simulink model "NetworkModelIntermediateIntersectionCRCA"  (R2018b)
settings: Solver=VariableStepAuto  StartTime=0.0  StopTime=10.0  RelTol=1e-3
values from neighbouring files (symbols this model uses):
  Ax = [0 1  0   0 ... (first row only)    [DroneSubsystemModelling.m]
  Ay = [0 1  0   0 ... (first row only)    [DroneSubsystemModelling.m]
  Bx = [0;0;0;b1]    [DroneSubsystemModelling.m]
  By = [0;0;0;b2]    [DroneSubsystemModelling.m]
  ConflictDrone1andDrone2 = ControlDetectionFunction(tout,PositionXDrone1TEST, PositionYDrone1TEST, PositionXDrone2TEST, PositionYDrone2TEST, ConflictDrone1andDrone2)    [ConflictDetectionTEST.m]
  ConflictDrone1andDrone3 = ControlDetectionFunction(tout,PositionXDrone1TEST, PositionYDrone1TEST, PositionXDrone3TEST, PositionYDrone3TEST, ConflictDrone1andDrone3)    [ConflictDetectionTEST.m]
  ConflictDrone1andDrone4 = ControlDetectionFunction(tout,PositionXDrone1TEST, PositionYDrone1TEST, PositionXDrone4TEST, PositionYDrone4TEST, ConflictDrone1andDrone4)    [ConflictDetectionTEST.m]
  ConflictDrone2andDrone3 = ControlDetectionFunction(tout,PositionXDrone2TEST, PositionYDrone2TEST, PositionXDrone3TEST, PositionYDrone3TEST, ConflictDrone2andDrone3)    [ConflictDetectionTEST.m]
  ConflictDrone2andDrone4 = ControlDetectionFunction(tout,PositionXDrone2, PositionYDrone2, PositionXDrone4, PositionYDrone4, ConflictDrone2andDrone4)    [ConflictDetection.m]    (also in ConflictDetectionTEST.m = ControlDetectionFunction(tout,PositionXDrone2TEST, PositionY)
  ConflictDrone3andDrone4 = ControlDetectionFunction(tout,PositionXDrone3TEST, PositionYDrone3TEST, PositionXDrone4TEST, PositionYDrone4TEST, ConflictDrone3andDrone4)    [ConflictDetectionTEST.m]
  ConflictDrone7andDrone8 = ControlDetectionFunction(tout,PositionXDrone7TEST, PositionYDrone7TEST, PositionXDrone8TEST, PositionYDrone8TEST, ConflictDrone7andDrone8)    [ConflictDetectionTEST.m]
  Cpx = [1 0 0 0]    [DroneSubsystemModelling.m]
  Cpy = [1 0 0 0]    [DroneSubsystemModelling.m]
  Cvx = [0 1 0 0]    [DroneSubsystemModelling.m]
  Cvy = [0 1 0 0]    [DroneSubsystemModelling.m]
  theta1 = -180    [MotionModelling.m]
  theta2 = -3*180/4    (= -135)    [MotionModelling.m]
  theta3 = -2*180/4    (= -90)    [MotionModelling.m]
  theta4 = -180/4    (= -45)    [MotionModelling.m]
  theta5 = 2*180    (= 360)    [MotionModelling.m]
  theta6 = 180/4    (= 45)    [MotionModelling.m]
  theta7 = 2*180/4    (= 90)    [MotionModelling.m]
  theta8 = 3*180/4    (= 135)    [MotionModelling.m]
  VelocityStarX1 = vx10    [MotionModelling.m]
  VelocityStarX2 = vx20    [MotionModelling.m]
  VelocityStarX3 = vx30    [MotionModelling.m]
  VelocityStarX4 = vx40    [MotionModelling.m]
  VelocityStarX5 = vx50    [MotionModelling.m]
  VelocityStarX6 = vx60    [MotionModelling.m]
  VelocityStarX7 = vx70    [MotionModelling.m]
  VelocityStarX8 = vx80    [MotionModelling.m]
  VelocityStarY1 = vy10    [MotionModelling.m]
  VelocityStarY2 = vy20    [MotionModelling.m]
  VelocityStarY3 = vy30    [MotionModelling.m]
  VelocityStarY4 = vy40    [MotionModelling.m]
  VelocityStarY5 = vy50    [MotionModelling.m]
  VelocityStarY6 = vy60    [MotionModelling.m]
  VelocityStarY7 = vy70    [MotionModelling.m]
  VelocityStarY8 = vy80    [MotionModelling.m]
  X10 = [x10 vx10 0 0]'    [MotionModelling.m]
  X20 = [x20 vx20 0 0]'    [MotionModelling.m]
  X30 = [x30 vx30 0 0]'    [MotionModelling.m]
  X40 = [x40 vx40 0 0]'    [MotionModelling.m]
  X50 = [x50 vx50 0 0]'    [MotionModelling.m]
  X60 = [x60 vx60 0 0]'    [MotionModelling.m]
  X70 = [x70 vx70 0 0]'    [MotionModelling.m]
  X80 = [x80 vx80 0 0]'    [MotionModelling.m]
  Y10 = [y10 vy10 0 0]'    [MotionModelling.m]
  Y20 = [y20 vy20 0 0]'    [MotionModelling.m]
  Y30 = [y30 vy30 0 0]'    [MotionModelling.m]
  Y40 = [y40 vy40 0 0]'    [MotionModelling.m]
  Y50 = [y50 vy50 0 0]'    [MotionModelling.m]
  Y60 = [y60 vy60 0 0]'    [MotionModelling.m]
  Y70 = [y70 vy70 0 0]'    [MotionModelling.m]
  Y80 = [y80 vy80 0 0]'    [MotionModelling.m]
undefined symbols (not defined in the file or in its folder): ConflictDrone5andDrone6, K
libraries: simulink x16
(part 1 of 2)
settings Model: Creator=CowUser  LastModifiedBy=CowUser
settings ConfigComp: DVTestSuiteOptimization=CombinedObjectives (Nonlinear Extended)  DVDetectOutOfBounds=on

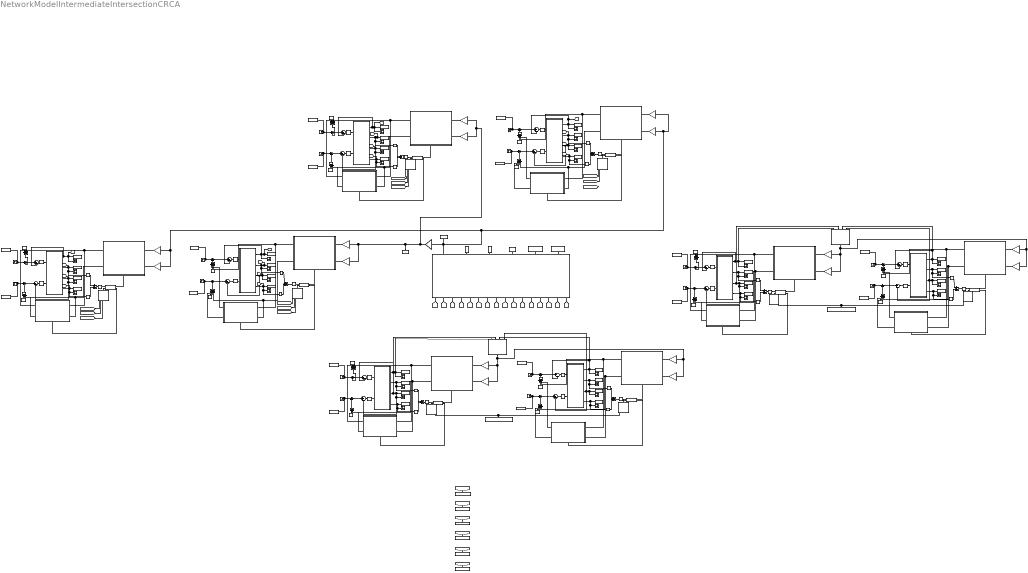
== system NetworkModelIntermediateIntersectionCRCA ==
  note: Drone 4
  note: Intermediate Intersection
      | (based on closure rate and closure angle)
      |
      | Right Hand Rule
  note: Drone 2
  note: Drone 5
  note: Drone 6
  note: Sample
  note: Drone 1
  note: Drone 3
  note: Drone 7
  note: Sample
  note: Drone 8
  note: Sample 4
  note: Sample 2
  note: Sample 6
  note: Sample 3
  note: Sample 5
  note: Sample 1
  Add{1..4,7,10..16,19..22} (16 alike) : Sum  Inputs=+++
  Add{5..6,8..9,17..18,23..24} (8 alike) : Sum
  Constant{1..4,6..8,10..14,16..19} (16 alike) : Constant  Value=0
  Constant20 : Constant  Value=ConflictDrone7andDrone8
  Constant25 : Constant  Value=ConflictDrone1andDrone3
  Constant26 : Constant  Value=ConflictDrone1andDrone2
  Constant27 : Constant  Value=ConflictDrone1andDrone4
  Constant28 : Constant  Value=ConflictDrone2andDrone4
  Constant29 : Constant  Value=ConflictDrone3andDrone4
  Constant30 : Constant  Value=ConflictDrone2andDrone3  VectorParams1D=off
  Constant5 : Constant  Value=ConflictDrone5andDrone6
  Drone1 Subsystem : Subsystem
  Drone2 Subsystem : Subsystem
  Drone2 Subsystem3 : Subsystem
  Drone3 Subsystem : Subsystem
  Drone4 Subsystem : Subsystem
  Drone4 Subsystem3 : Subsystem
  Drone5 Subsystem : Subsystem
  Drone6 Subsystem : Subsystem
  Gain : Gain  Gain=K
  Gain1 : Gain  Gain=-sind (theta4)
  Gain10 : Gain  Gain=cosd (theta1)
  Gain11 : Gain  Gain=-cosd (theta3)
  Gain12 : Gain  Gain=sind (theta1)
  Gain13 : Gain  Gain=-sind (theta8)
  Gain14 : Gain  Gain=cosd (theta7)
  Gain15 : Gain  Gain=-cosd (theta8)
  Gain16 : Gain  Gain=sind (theta7)
  Gain2 : Gain  Gain=cosd (theta2)
  Gain3 : Gain  Gain=-cosd (theta4)
  Gain4 : Gain  Gain=sind (theta2)
  Gain5 : Gain  Gain=-sind (theta6)
  Gain6 : Gain  Gain=cosd (theta5)
  Gain7 : Gain  Gain=-cosd (theta6)
  Gain8 : Gain  Gain=sind (theta5)
  Gain9 : Gain  Gain=-sind (theta3)
  If Action Subsystem1 : Subsystem  TreatAsAtomicUnit=on
  If Action Subsystem2 : Subsystem  TreatAsAtomicUnit=on
  If Action Subsystem3 : Subsystem  TreatAsAtomicUnit=on
  If Action Subsystem4 : Subsystem  TreatAsAtomicUnit=on
  If Action Subsystem5 : Subsystem  TreatAsAtomicUnit=on
  If Action Subsystem6 : Subsystem  TreatAsAtomicUnit=on
  If Action Subsystem7 : Subsystem  TreatAsAtomicUnit=on
  If Action Subsystem8 : Subsystem  TreatAsAtomicUnit=on
  If{1..8} (8 alike) : If  NumInputs=2  IfExpression=(u1 <= R)&(u2 == 1)  ElseIfExpressions=(u1 > R)&(u2 == 1)  ShowElse=off
  MATLAB Function1 : MATLAB Function  TreatAsAtomicUnit=on
  MATLAB Function2 : MATLAB Function  TreatAsAtomicUnit=on
  MATLAB Function3 : MATLAB Function  TreatAsAtomicUnit=on
  OR{1..8} (8 alike) : Logic  Operator=OR  Inputs=7  IconShape=distinctive  AllPortsSameDT=off  OutDataTypeStr='double'
  PID Controller{1..16} (16 alike) : simulink/Continuous/PID Controller  Controller=PID  Form=Parallel  TimeDomain=Continuous-time  SampleTime=-1  IntegratorMethod=Forward Euler  FilterMethod=Forward Euler  ControllerParametersSource=internal  P=1.97139727738968e-05  I=1.5233344900537e-08  D=0.00566857635684116  UseFilter=on  N=15.1370363747334  TunerSelectOption=Transfer Function Based (PID Tuner App)  InitialConditionSource=internal  InitialConditionForIntegrator=0  InitialConditionForFilter=0  DifferentiatorICPrevScaledInput=0  ExternalReset=none  TrackingMode=off  Kt=1  LimitOutput=off  UpperSaturationLimit=inf  LowerSaturationLimit=-inf  LinearizeAsGain=on  AntiWindupMode=none  Kb=1  POutMin=[]  POutMax=[]  IOutMin=[]  IOutMax=[]  DOutMin=[]  DOutMax=[]  NOutMin=[]  NOutMax=[]  SumOutMin=[]  SumOutMax=[]  SaturationOutMin=[]  SaturationOutMax=[]  PParamMin=[]  PParamMax=[]  IParamMin=[]  IParamMax=[]  DParamMin=[]  DParamMax=[]  NParamMin=[]  NParamMax=[]  KbParamMin=[]  KbParamMax=[]  KtParamMin=[]  KtParamMax=[]  KbOutMin=[]  KbOutMax=[]  KtOutMin=[]  KtOutMax=[]  IntegratorOutMin=[]  IntegratorOutMax=[]  FilterOutMin=[]  FilterOutMax=[]  SumI1OutMin=[]  SumI1OutMax=[]  SumI2OutMin=[]  SumI2OutMax=[]  SumI3OutMin=[]  SumI3OutMax=[]  SumI4OutMin=[]  SumI4OutMax=[]  SumDOutMin=[]  SumDOutMax=[]  DifferentiatorOutMin=[]  DifferentiatorOutMax=[]  FilterDiffOutCoefMin=[]  FilterDiffOutCoefMax=[]  ReciprocalOutMin=[]  ReciprocalOutMax=[]  SumDenOutMin=[]  SumDenOutMax=[]  SumNumOutMin=[]  SumNumOutMax=[]  DivideOutMin=[]  DivideOutMax=[]  IntegratorContinuousStateAttributes=''  IntegratorStateMustResolveToSignalObject=off  IntegratorRTWStateStorageClass=Auto  FilterContinuousStateAttributes=''  FilterStateMustResolveToSignalObject=off  FilterRTWStateStorageClass=Auto  ParallelPVariant=InternalParameters  IdealPVariant=Disabled  IVariant=InternalParameters  DVariant=InternalParameters  IntegratorVariant=Continuous  SatVariant=Disabled  AWVariant=Passthrough  PCopyVariant=Disabled  TRVariant=Disabled  FdbkBlocksVariant=Forward  IdealPFdbkVariant=Disabled  SatFdbkVariant=Disabled  DerivativeFilterVariant=ContFilter  NVariant=InternalParameters  NCopyVariant=Disabled  FilterICVariant=InternalICsFilter  IntegratorICVariant=InternalICs  ExternalResetVariant=Disabled  TRSumVariant=Passthrough  SumFdbkVariant=Disabled  SumVariant=Sum_PID
  PositionXDrone{1,3,5..8,11,44} (8 alike) : Scope
  PositionYDrone{1,3,5..8,11,44} (8 alike) : Scope
  Sqrt{1..8} (8 alike) : Sqrt  SaturateOnIntegerOverflow=on
  Square{1..16} (16 alike) : Math  Operator=square  SaturateOnIntegerOverflow=on
  Step 1 : Step  Time=0  After=VelocityStarX5  SampleTime=0
  Step 10 : Step  Time=0  After=VelocityStarY1  SampleTime=0
  Step 11 : Step  Time=0  After=VelocityStarX3  SampleTime=0
  Step 12 : Step  Time=0  After=VelocityStarY3  SampleTime=0
  Step 13 : Step  Time=0  After=VelocityStarX7  SampleTime=0
  Step 14 : Step  Time=0  After=VelocityStarY7  SampleTime=0
  Step 15 : Step  Time=0  After=VelocityStarX8  SampleTime=0
  Step 16 : Step  Time=0  After=VelocityStarY8  SampleTime=0
  Step 2 : Step  Time=0  After=VelocityStarY5  SampleTime=0
  Step 3 : Step  Time=0  After=VelocityStarX2  SampleTime=0
  Step 4 : Step  Time=0  After=VelocityStarY2  SampleTime=0
  Step 5 : Step  Time=0  After=VelocityStarX4  SampleTime=0
  Step 6 : Step  Time=0  After=VelocityStarY4  SampleTime=0
  Step 7 : Step  Time=0  After=VelocityStarX6  SampleTime=0
  Step 8 : Step  Time=0  After=VelocityStarY6  SampleTime=0
  Step 9 : Step  Time=0  After=VelocityStarX1  SampleTime=0
  Sum{1..32} (32 alike) : Sum  Inputs=|+-
  Switch Case Action Subsystem : Subsystem  TreatAsAtomicUnit=on
  Switch Case Action Subsystem1 : Subsystem  TreatAsAtomicUnit=on
  Switch Case Action Subsystem2 : Subsystem  TreatAsAtomicUnit=on
  Switch Case Action Subsystem3 : Subsystem  TreatAsAtomicUnit=on
  Switch Case Action Subsystem4 : Subsystem  TreatAsAtomicUnit=on
  Switch Case Action Subsystem5 : Subsystem  TreatAsAtomicUnit=on
  Switch Case Action Subsystem6 : Subsystem  TreatAsAtomicUnit=on
  Switch Case Action Subsystem7 : Subsystem  TreatAsAtomicUnit=on
  To Workspace : ToWorkspace  VariableName=Vdiff2  SampleTime=-1
  To Workspace1 : ToWorkspace  VariableName=VelocityYDrone6  SampleTime=-1
  To Workspace10 : ToWorkspace  VariableName=VelocityYDrone4  SampleTime=-1
  To Workspace11 : ToWorkspace  VariableName=PositionXDrone4  SampleTime=-1
  To Workspace12 : ToWorkspace  VariableName=VelocityXDrone4  SampleTime=-1
  To Workspace13 : ToWorkspace  VariableName=VelocityStarX4  SampleTime=-1
  To Workspace14 : ToWorkspace  VariableName=PositionYDrone4  SampleTime=-1
  To Workspace15 : ToWorkspace  VariableName=PositionXDrone2  SampleTime=-1
  To Workspace16 : ToWorkspace  VariableName=VelocityXDrone2  SampleTime=-1
  To Workspace17 : ToWorkspace  VariableName=VelocityStarX2  SampleTime=-1
  To Workspace18 : ToWorkspace  VariableName=PositionYDrone2  SampleTime=-1
  To Workspace19 : ToWorkspace  VariableName=VelocityXDrone5  SampleTime=-1
  To Workspace2 : ToWorkspace  VariableName=PositionXDrone6  SampleTime=-1
  To Workspace20 : ToWorkspace  VariableName=VelocityStarX5  SampleTime=-1
  To Workspace21 : ToWorkspace  VariableName=PositionYDrone5  SampleTime=-1
  To Workspace22 : ToWorkspace  VariableName=VelocityStarY5  SampleTime=-1
  To Workspace23 : ToWorkspace  VariableName=VelocityStarY6  SampleTime=-1
  To Workspace24 : ToWorkspace  VariableName=VelocityYDrone5  SampleTime=-1
  To Workspace25 : ToWorkspace  VariableName=VelocityYDrone3  SampleTime=-1
  To Workspace26 : ToWorkspace  VariableName=VelocityXDrone1  SampleTime=-1
  To Workspace27 : ToWorkspace  VariableName=PositionXDrone3  SampleTime=-1
  To Workspace28 : ToWorkspace  VariableName=VelocityStarX1  SampleTime=-1
  To Workspace29 : ToWorkspace  VariableName=PositionYDrone1  SampleTime=-1
  To Workspace3 : ToWorkspace  VariableName=VelocityXDrone6  SampleTime=-1
  To Workspace30 : ToWorkspace  VariableName=VelocityStarY1  SampleTime=-1
  To Workspace31 : ToWorkspace  VariableName=VelocityStarY3  SampleTime=-1
  To Workspace32 : ToWorkspace  VariableName=VelocityYDrone1  SampleTime=-1
  To Workspace33 : ToWorkspace  VariableName=VelocityXDrone3  SampleTime=-1
  To Workspace34 : ToWorkspace  VariableName=VelocityStarX3  SampleTime=-1
  To Workspace35 : ToWorkspace  VariableName=PositionYDrone3  SampleTime=-1
  To Workspace36 : ToWorkspace  VariableName=PositionXDrone1  SampleTime=-1
  To Workspace37 : ToWorkspace  VariableName=VelocityYDrone8  SampleTime=-1
  To Workspace38 : ToWorkspace  VariableName=VelocityXDrone7  SampleTime=-1
  To Workspace39 : ToWorkspace  VariableName=PositionXDrone8  SampleTime=-1
  To Workspace4 : ToWorkspace  VariableName=VelocityStarX6  SampleTime=-1
  To Workspace40 : ToWorkspace  VariableName=VelocityStarX7  SampleTime=-1
  To Workspace41 : ToWorkspace  VariableName=PositionYDrone7  SampleTime=-1
  To Workspace42 : ToWorkspace  VariableName=VelocityStarY7  SampleTime=-1
  To Workspace43 : ToWorkspace  VariableName=VelocityStarY8  SampleTime=-1
  To Workspace44 : ToWorkspace  VariableName=VelocityYDrone7  SampleTime=-1
  To Workspace45 : ToWorkspace  VariableName=VelocityXDrone8  SampleTime=-1
  To Workspace46 : ToWorkspace  VariableName=VelocityStarX8  SampleTime=-1
  To Workspace47 : ToWorkspace  VariableName=PositionYDrone8  SampleTime=-1
  To Workspace48 : ToWorkspace  VariableName=PositionXDrone7  SampleTime=-1
  To Workspace49 : ToWorkspace  VariableName=Vdiff1  SampleTime=-1
  To Workspace5 : ToWorkspace  VariableName=PositionYDrone6  SampleTime=-1
  To Workspace50 : ToWorkspace  VariableName=N  SampleTime=-1
  To Workspace51 : ToWorkspace  VariableName=M  SampleTime=-1
  To Workspace52 : ToWorkspace  VariableName=RANGE  SampleTime=-1
  To Workspace53 : ToWorkspace  VariableName=minimumClosureTime  SampleTime=-1
  To Workspace54 : ToWorkspace  VariableName=numOfCollisions  SampleTime=-1
  To Workspace6 : ToWorkspace  VariableName=PositionXDrone5  SampleTime=-1
  To Workspace7 : ToWorkspace  VariableName=VelocityStarY2  SampleTime=-1
  To Workspace8 : ToWorkspace  VariableName=VelocityStarY4  SampleTime=-1
  To Workspace9 : ToWorkspace  VariableName=VelocityYDrone2  SampleTime=-1
  VelocityXDrone{1,3,5..8,11,44} (8 alike) : Scope
  VelocityYDrone{1,3,5..8,11,44} (8 alike) : Scope
  wires:
  Switch Case Action Subsystem1/1(dVx4) -> Add12/1
  Drone4 Subsystem/3(Vy) -> Sum17/2, [qDotyD], VelocityYDrone44/1, To Workspace10/1
  OR4/1 -> If4/2
  Drone2 Subsystem/4(y) -> [qyB], To Workspace18/1, Square9/1, PositionYDrone11/1
  Drone2 Subsystem/1(Vx) -> Sum15/2, [qDotxB], VelocityXDrone11/1, To Workspace16/1
  If Action Subsystem3/1(dVx4) -> Switch Case Action Subsystem1/1(deltaVx4), Add12/3
  If Action Subsystem2/1(dVx2) -> Switch Case Action Subsystem/1(deltaVx2), Add11/3
  Gain1/1 -> If Action Subsystem3/2(deltaVy4)
  PID Controller4/1 -> Drone4 Subsystem/2("InputForceY* ")
  Gain/1 -> Gain4/1, Gain2/1, Gain9/1, Gain11/1, To Workspace/1
  If4/1 -> If Action Subsystem2/Action
  Add12/1 -> Sum18/2
  Sqrt4/1 -> If4/1
  Sum18/1 -> Sum16/1
  Drone4 Subsystem/2(x) -> Square10/1, PositionXDrone44/1, To Workspace11/1, [qxD]
  Add9/1 -> Sqrt5/1
  Switch Case Action Subsystem/2(dVy2) -> Add10/3
  Add8/1 -> Sqrt4/1
  If2/1 -> If Action Subsystem3/Action
  PID Controller8/1 -> Drone2 Subsystem/1(InputForceX*)
  Sum15/1 -> PID Controller8/1
  If4/2 -> Switch Case Action Subsystem/Action
  Square9/1 -> Add8/2
  Add13/1 -> Sum19/2
  OR3/1 -> If2/2
  Square11/1 -> Add9/2
  PID Controller2/1 -> Drone2 Subsystem/2("InputForceY* ")
  Constant12/1 -> Add12/2
  Square8/1 -> Add8/1
  PID Controller5/1 -> Drone4 Subsystem/1(InputForceX*)
  Constant13/1 -> Add13/2
  If2/2 -> Switch Case Action Subsystem1/Action
  Sum17/1 -> PID Controller4/1
  Sum20/1 -> Sum15/1
  Step 5/1 -> Sum18/1, To Workspace13/1
  Step 4/1 -> Sum14/1, To Workspace7/1
  Sum16/1 -> PID Controller5/1
  Sqrt5/1 -> If2/1
  Sum13/1 -> PID Controller2/1
  Add11/1 -> Sum20/2
  Switch Case Action Subsystem1/2(dVy4) -> Add13/1
  Constant10/1 -> Add11/2
  Switch Case Action Subsystem/1(dVx2) -> Add11/1
  If Action Subsystem2/2(dVy2) -> Add10/2, Switch Case Action Subsystem/2(deltaVy2)
  Sum14/1 -> Sum13/1
  If Action Subsystem3/2(dVy4) -> Switch Case Action Subsystem1/2(deltaVy4), Add13/3
  Add10/1 -> Sum14/2
  Constant11/1 -> Add10/1
  Drone4 Subsystem/1(Vx) -> [qDotxD], Sum16/2, To Workspace12/1, VelocityXDrone44/1
  Gain2/1 -> If Action Subsystem2/1(deltaVx2)
  Gain3/1 -> If Action Subsystem3/1(deltaVx4)
  Drone4 Subsystem/4(y) -> [qyD], Square11/1, PositionYDrone44/1, To Workspace14/1
  Gain4/1 -> If Action Subsystem2/2(deltaVy2)
  Drone2 Subsystem/3(Vy) -> [qDotyB], To Workspace9/1, Sum13/2, VelocityYDrone11/1
  Step 3/1 -> Sum20/1, To Workspace17/1
  Sum19/1 -> Sum17/1
  Square10/1 -> Add9/1
  Step 6/1 -> To Workspace8/1, Sum19/1
  Sum7/1 -> Sum5/1
  Step 1/1 -> Sum8/1, To Workspace20/1
  Drone5 Subsystem/3(Vy) -> To Workspace24/1, Sum1/2, VelocityYDrone5/1, MATLAB Function1/2(qDotxj)
  Drone6 Subsystem/4(y) -> Square2/1, PositionYDrone6/1, To Workspace5/1
  Gain7/1 -> If Action Subsystem4/1(deltaVx6)
  Drone6 Subsystem/1(Vx) -> MATLAB Function1/3(qDotyi), Sum4/2, To Workspace3/1, VelocityXDrone6/1
  Add1/1 -> Sum2/2
  If Action Subsystem4/2(dVy6) -> Switch Case Action Subsystem3/2(deltaVy6), Add4/3
  Sum2/1 -> Sum1/1
  If Action Subsystem1/2(dVy5) -> Add1/2, Switch Case Action Subsystem2/2(deltaVy5)
  Sum1/1 -> PID Controller1/1
  Switch Case Action Subsystem3/2(dVy6) -> Add4/1
  Switch Case Action Subsystem2/1(dVx5) -> Add2/1
  Add2/1 -> Sum8/2
  Gain6/1 -> If Action Subsystem1/1(deltaVx5)
  Sqrt2/1 -> If1/1
  Sum4/1 -> PID Controller6/1
  Sum5/1 -> PID Controller3/1
  If1/2 -> Switch Case Action Subsystem3/Action
  Step 7/1 -> Sum6/1, To Workspace4/1
  Step 2/1 -> Sum2/1, To Workspace22/1
  Square3/1 -> Add5/1
  Square4/1 -> Add5/2
  Add4/1 -> Sum7/2
  PID Controller7/1 -> Drone5 Subsystem/1(InputForceX*)
  Sum8/1 -> Sum3/1
  If3/2 -> Switch Case Action Subsystem2/Action
  Sum3/1 -> PID Controller7/1
  If1/1 -> If Action Subsystem4/Action
  Constant1/1 -> Add2/2
  PID Controller6/1 -> Drone6 Subsystem/1(InputForceX*)
  Add3/1 -> Sum6/2
  PID Controller1/1 -> Drone5 Subsystem/2("InputForceY* ")
  Drone6 Subsystem/2(x) -> Square1/1, PositionXDrone6/1, To Workspace2/1
  PID Controller3/1 -> Drone6 Subsystem/2("InputForceY* ")
  Square2/1 -> Add6/2
  Sum6/1 -> Sum4/1
  If Action Subsystem4/1(dVx6) -> Switch Case Action Subsystem3/1(deltaVx6), Add3/3
  Add6/1 -> Sqrt2/1
  Step 8/1 -> To Workspace23/1, Sum7/1
  Gain8/1 -> If Action Subsystem1/2(deltaVy5)
  Drone5 Subsystem/1(Vx) -> Sum3/2, MATLAB Function1/1(qDotxi), VelocityXDrone5/1, To Workspace19/1
  Switch Case Action Subsystem2/2(dVy5) -> Add1/3
  If Action Subsystem1/1(dVx5) -> Switch Case Action Subsystem2/1(deltaVx5), Add2/3
  Drone6 Subsystem/3(Vy) -> MATLAB Function1/4(qDotyj), Sum5/2, VelocityYDrone6/1, To Workspace1/1
  If3/1 -> If Action Subsystem1/Action
  Constant5/1 -> OR1/1, OR2/7
  MATLAB Function1/1(y) -> Gain8/1, Gain6/1, Gain7/1, Gain5/1
  Sqrt1/1 -> If3/1
  Add5/1 -> Sqrt1/1
  OR2/1 -> If3/2
  Square1/1 -> Add6/1
  Drone5 Subsystem/4(y) -> To Workspace21/1, Square4/1, PositionYDrone5/1
  Constant2/1 -> Add1/1
  Gain5/1 -> If Action Subsystem4/2(deltaVy6)
  OR1/1 -> If1/2
  Constant3/1 -> Add3/2
  Switch Case Action Subsystem3/1(dVx6) -> Add3/1
  Constant4/1 -> Add4/2
  Drone5 Subsystem/2(x) -> Square3/1, PositionXDrone5/1, To Workspace6/1
  Switch Case Action Subsystem5/1(dVx3) -> Add15/1
  Constant8/1 -> Add15/2
  OR5/1 -> If5/2
  Drone1 Subsystem/4(y) -> [qyA], To Workspace29/1, Square12/1, PositionYDrone1/1
  Square5/1 -> Add18/1
  Gain9/1 -> If Action Subsystem6/2(deltaVy3)
  Add17/1 -> Sqrt3/1
  Sqrt3/1 -> If6/1
  Drone3 Subsystem/3(Vy) -> Sum21/2, [qDotyC], VelocityYDrone3/1, To Workspace25/1
  Drone1 Subsystem/1(Vx) -> [qDotxA], VelocityXDrone1/1, To Workspace26/1, Sum11/2
  Gain12/1 -> If Action Subsystem5/2(deltaVy1)
  Step 12/1 -> To Workspace31/1, Sum23/1
  Switch Case Action Subsystem4/2(dVy1) -> Add7/3
  If6/1 -> If Action Subsystem5/Action
  If Action Subsystem6/1(dVx3) -> Switch Case Action Subsystem5/1(deltaVx3), Add15/3
  Sum22/1 -> Sum12/1
  Square6/1 -> Add18/2
  PID Controller10/1 -> Drone3 Subsystem/2("InputForceY* ")
  Drone3 Subsystem/2(x) -> Square5/1, PositionXDrone3/1, [qxC], To Workspace27/1
  If6/2 -> Switch Case Action Subsystem4/Action
  Add15/1 -> Sum22/2
  Constant7/1 -> Add7/1
  Sum11/1 -> PID Controller12/1
  Sum9/1 -> PID Controller9/1
  Step 10/1 -> Sum10/1, To Workspace30/1
  Add18/1 -> Sqrt6/1
  Switch Case Action Subsystem5/2(dVy3) -> Add16/1
  If5/2 -> Switch Case Action Subsystem5/Action
  Drone3 Subsystem/1(Vx) -> Sum12/2, [qDotxC], To Workspace33/1, VelocityXDrone3/1
  Gain11/1 -> If Action Subsystem6/1(deltaVx3)
  If Action Subsystem5/2(dVy1) -> Add7/2, Switch Case Action Subsystem4/2(deltaVy1)
  If Action Subsystem5/1(dVx1) -> Switch Case Action Subsystem4/1(deltaVx1), Add14/3
  OR6/1 -> If6/2
  Sum12/1 -> PID Controller11/1
  Step 11/1 -> Sum22/1, To Workspace34/1
  Add7/1 -> Sum10/2
  Sum21/1 -> PID Controller10/1
  PID Controller9/1 -> Drone1 Subsystem/2("InputForceY* ")
  If5/1 -> If Action Subsystem6/Action
  Gain10/1 -> If Action Subsystem5/1(deltaVx1)
  PID Controller11/1 -> Drone3 Subsystem/1(InputForceX*)
  Drone3 Subsystem/4(y) -> [qyC], Square6/1, PositionYDrone3/1, To Workspace35/1
  Drone1 Subsystem/3(Vy) -> [qDotyA], To Workspace32/1, Sum9/2, VelocityYDrone1/1
  MATLAB Function2/1(Vdiff) -> Gain3/1, Gain1/1, Gain12/1, Gain10/1, To Workspace49/1, Gain/1
  Step 9/1 -> Sum24/1, To Workspace28/1
  Constant6/1 -> Add14/2
  Square12/1 -> Add17/2
  Sum10/1 -> Sum9/1
  Add14/1 -> Sum24/2
  Square7/1 -> Add17/1
  Constant14/1 -> Add16/2
  Sqrt6/1 -> If5/1
  Add16/1 -> Sum23/2
  Sum24/1 -> Sum11/1
  PID Controller12/1 -> Drone1 Subsystem/1(InputForceX*)
  Switch Case Action Subsystem4/1(dVx1) -> Add14/1
  If Action Subsystem6/2(dVy3) -> Switch Case Action Subsystem5/2(deltaVy3), Add16/3
  Sum23/1 -> Sum21/1
  Switch Case Action Subsystem7/1(dVx4) -> Add21/1
  Constant18/1 -> Add21/2
  OR7/1 -> If7/2
  Drone2 Subsystem3/4(y) -> To Workspace41/1, Square16/1, PositionYDrone7/1
  Square13/1 -> Add24/1
  Gain13/1 -> If Action Subsystem8/2(deltaVy8)
  Add23/1 -> Sqrt7/1
  Sqrt7/1 -> If8/1
  Drone4 Subsystem3/3(Vy) -> MATLAB Function3/4(qDotyj), Sum29/2, VelocityYDrone8/1, To Workspace37/1
  Drone2 Subsystem3/1(Vx) -> Sum27/2, MATLAB Function3/1(qDotxi), VelocityXDrone7/1, To Workspace38/1
  Gain16/1 -> If Action Subsystem7/2(deltaVy7)
  Step 16/1 -> To Workspace43/1, Sum31/1
  Switch Case Action Subsystem6/2(dVy7) -> Add19/3
  If8/1 -> If Action Subsystem7/Action
  If Action Subsystem8/1(dVx8) -> Switch Case Action Subsystem7/1(deltaVx4), Add21/3
  Sum30/1 -> Sum28/1
  Square14/1 -> Add24/2
  PID Controller14/1 -> Drone4 Subsystem3/2("InputForceY* ")
  Drone4 Subsystem3/2(x) -> Square13/1, PositionXDrone8/1, To Workspace39/1
  If8/2 -> Switch Case Action Subsystem6/Action
  Drone2 Subsystem3/2(x) -> Square15/1, PositionXDrone7/1, To Workspace48/1
  Add21/1 -> Sum30/2
  Constant17/1 -> Add19/1
  Sum27/1 -> PID Controller16/1
  Sum25/1 -> PID Controller13/1
  Step 14/1 -> Sum26/1, To Workspace42/1
  Add24/1 -> Sqrt8/1
  Switch Case Action Subsystem7/2(dVy4) -> Add22/1
  If7/2 -> Switch Case Action Subsystem7/Action
  Constant20/1 -> OR7/1, OR8/7
  Drone4 Subsystem3/1(Vx) -> MATLAB Function3/3(qDotyi), Sum28/2, To Workspace45/1, VelocityXDrone8/1
  Gain15/1 -> If Action Subsystem8/1(deltaVx8)
  If Action Subsystem7/2(dVy7) -> Add19/2, Switch Case Action Subsystem6/2(deltaVy7)
  If Action Subsystem7/1(dVx7) -> Switch Case Action Subsystem6/1(deltaVx7), Add20/3
  OR8/1 -> If8/2
  Sum28/1 -> PID Controller15/1
  Step 15/1 -> Sum30/1, To Workspace46/1
  Add19/1 -> Sum26/2
  Sum29/1 -> PID Controller14/1
  PID Controller13/1 -> Drone2 Subsystem3/2("InputForceY* ")
  If7/1 -> If Action Subsystem8/Action
  Gain14/1 -> If Action Subsystem7/1(deltaVx7)
  PID Controller15/1 -> Drone4 Subsystem3/1(InputForceX*)
  Drone4 Subsystem3/4(y) -> Square14/1, PositionYDrone8/1, To Workspace47/1
  Drone2 Subsystem3/3(Vy) -> To Workspace44/1, Sum25/2, VelocityYDrone7/1, MATLAB Function3/2(qDotxj)
  MATLAB Function3/1(y) -> Gain16/1, Gain14/1, Gain15/1, Gain13/1
  Step 13/1 -> Sum32/1, To Workspace40/1
  Constant16/1 -> Add20/2
  Square16/1 -> Add23/2
  Sum26/1 -> Sum25/1
  Add20/1 -> Sum32/2
  Square15/1 -> Add23/1
  Constant19/1 -> Add22/2
  Sqrt8/1 -> If7/1
  Add22/1 -> Sum31/2
  Sum32/1 -> Sum27/1
  PID Controller16/1 -> Drone2 Subsystem3/1(InputForceX*)
  Switch Case Action Subsystem6/1(dVx7) -> Add20/1
  If Action Subsystem8/2(dVy8) -> Switch Case Action Subsystem7/2(deltaVy4), Add22/3
  Sum31/1 -> Sum29/1
  Drone1 Subsystem/2(x) -> [qxA], Square7/1, PositionXDrone1/1, To Workspace36/1
  Drone2 Subsystem/2(x) -> [qxB], To Workspace15/1, Square8/1, PositionXDrone11/1
  [qxA] -> MATLAB Function2/1(qxA)
  [qxB] -> MATLAB Function2/2(qxB)
  [qxC] -> MATLAB Function2/3(qxC)
  [qxD] -> MATLAB Function2/4(qxD)
  [qyA] -> MATLAB Function2/5(qyA)
  [qyB] -> MATLAB Function2/6(qyB)
  [qyC] -> MATLAB Function2/7(qyC)
  [qyD] -> MATLAB Function2/8(qyD)
  [qDotyC] -> MATLAB Function2/15(qDotyC)
  [qDotyB] -> MATLAB Function2/14(qDotyB)
  [qDotyD] -> MATLAB Function2/16(qDotyD)
  [qDotxB] -> MATLAB Function2/10(qDotxB)
  [qDotxC] -> MATLAB Function2/11(qDotxC)
  [qDotyA] -> MATLAB Function2/13(qDotyA)
  [qDotxA] -> MATLAB Function2/9(qDotxA)
  [qDotxD] -> MATLAB Function2/12(qDotxD)
  MATLAB Function2/2(M) -> To Workspace51/1
  MATLAB Function2/3(N) -> To Workspace50/1
  MATLAB Function2/4(RANGE) -> To Workspace52/1
  MATLAB Function2/5(minimumClosureTime) -> To Workspace53/1
  MATLAB Function2/6(numOfCollisions) -> To Workspace54/1
  [ConflictDrone1andDrone3] -> OR6/1
  [ConflictDrone1andDrone2] -> OR6/2
  [ConflictDrone1andDrone4] -> OR6/3
  [ConflictDrone1andDrone3] -> OR5/1
  [ConflictDrone2andDrone3] -> OR5/2
  [ConflictDrone3andDrone4] -> OR5/3
  [ConflictDrone1andDrone2] -> OR4/1
  [ConflictDrone2andDrone3] -> OR4/2
  [ConflictDrone2andDrone4] -> OR4/3
  [ConflictDrone1andDrone4] -> OR3/1
  [ConflictDrone2andDrone4] -> OR3/2
  Constant27/1 -> [ConflictDrone1andDrone4]
  Constant29/1 -> [ConflictDrone3andDrone4]
  Constant25/1 -> [ConflictDrone1andDrone3]
  Constant30/1 -> [ConflictDrone2andDrone3]
  Constant28/1 -> [ConflictDrone2andDrone4]
  Constant26/1 -> [ConflictDrone1andDrone2]

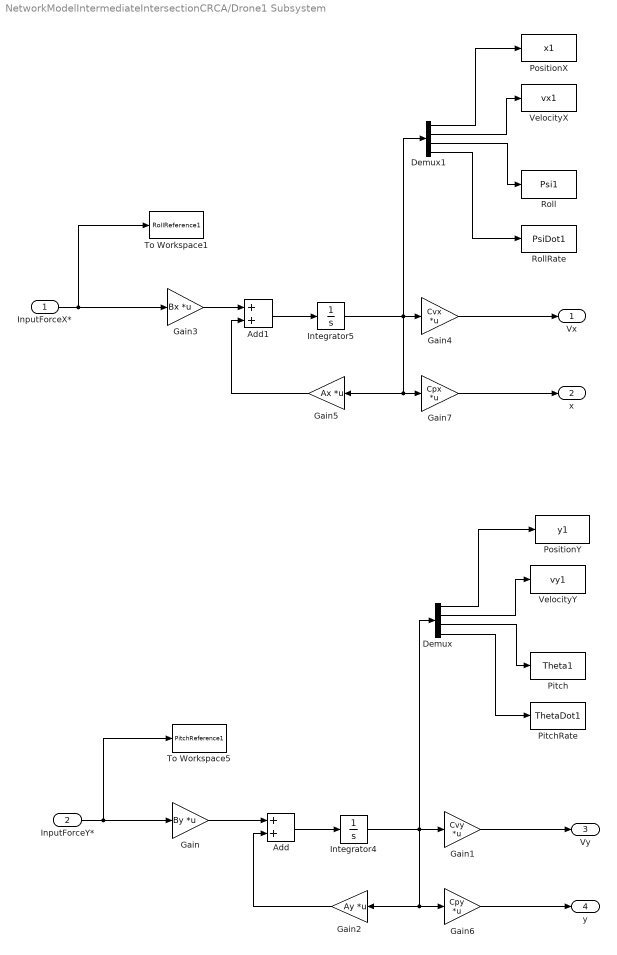
== system NetworkModelIntermediateIntersectionCRCA/Drone1 Subsystem ==
  InputForceX* : Inport
  "InputForceY* " : Inport  Port=2
  Add : Sum
  Add1 : Sum
  Demux : Demux
  Demux1 : Demux
  Gain : Gain  Gain=By  Multiplication=Matrix(K*u)
  Gain1 : Gain  Gain=Cvy  Multiplication=Matrix(K*u)
  Gain2 : Gain  Gain=Ay  Multiplication=Matrix(K*u)
  Gain3 : Gain  Gain=Bx  Multiplication=Matrix(K*u)
  Gain4 : Gain  Gain=Cvx  Multiplication=Matrix(K*u)
  Gain5 : Gain  Gain=Ax  Multiplication=Matrix(K*u)
  Gain6 : Gain  Gain=Cpy  Multiplication=Matrix(K*u)
  Gain7 : Gain  Gain=Cpx  Multiplication=Matrix(K*u)
  Integrator4 : Integrator  InitialCondition=Y10
  Integrator5 : Integrator  InitialCondition=X10
  Pitch : ToWorkspace  VariableName=Theta1  SampleTime=-1
  PitchRate : ToWorkspace  VariableName=ThetaDot1  SampleTime=-1
  PositionX : ToWorkspace  VariableName=x1  SampleTime=-1
  PositionY : ToWorkspace  VariableName=y1  SampleTime=-1
  Roll : ToWorkspace  VariableName=Psi1  SampleTime=-1
  RollRate : ToWorkspace  VariableName=PsiDot1  SampleTime=-1
  To Workspace1 : ToWorkspace  VariableName=RollReference1  SampleTime=-1
  To Workspace5 : ToWorkspace  VariableName=PitchReference1  SampleTime=-1
  VelocityX : ToWorkspace  VariableName=vx1  SampleTime=-1
  VelocityY : ToWorkspace  VariableName=vy1  SampleTime=-1
  Vx : Outport
  x : Outport  Port=2
  Vy : Outport  Port=3
  y : Outport  Port=4
  wires:
  Demux/1 -> PositionY/1
  Demux1/2 -> VelocityX/1
  Demux1/4 -> RollRate/1
  Demux1/3 -> Roll/1
  Gain4/1 -> Vx/1
  "InputForceY* "/1 -> Gain/1, To Workspace5/1
  Gain/1 -> Add/1
  Demux/4 -> PitchRate/1
  Demux/3 -> Pitch/1
  Add/1 -> Integrator4/1
  Demux1/1 -> PositionX/1
  Gain1/1 -> Vy/1
  InputForceX*/1 -> Gain3/1, To Workspace1/1
  Gain7/1 -> x/1
  Integrator4/1 -> Gain6/1, Gain2/1, Demux/1, Gain1/1
  Demux/2 -> VelocityY/1
  Gain6/1 -> y/1
  Gain3/1 -> Add1/1
  Add1/1 -> Integrator5/1
  Gain2/1 -> Add/2
  Integrator5/1 -> Gain4/1, Gain5/1, Gain7/1, Demux1/1
  Gain5/1 -> Add1/2

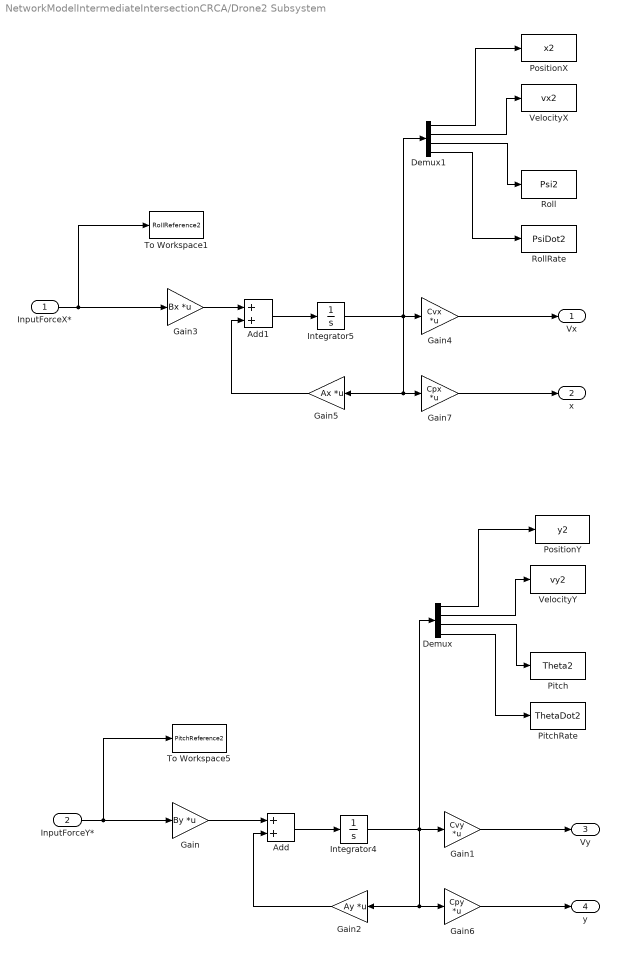
== system NetworkModelIntermediateIntersectionCRCA/Drone2 Subsystem ==
  InputForceX* : Inport
  "InputForceY* " : Inport  Port=2
  Add : Sum
  Add1 : Sum
  Demux : Demux
  Demux1 : Demux
  Gain : Gain  Gain=By  Multiplication=Matrix(K*u)
  Gain1 : Gain  Gain=Cvy  Multiplication=Matrix(K*u)
  Gain2 : Gain  Gain=Ay  Multiplication=Matrix(K*u)
  Gain3 : Gain  Gain=Bx  Multiplication=Matrix(K*u)
  Gain4 : Gain  Gain=Cvx  Multiplication=Matrix(K*u)
  Gain5 : Gain  Gain=Ax  Multiplication=Matrix(K*u)
  Gain6 : Gain  Gain=Cpy  Multiplication=Matrix(K*u)
  Gain7 : Gain  Gain=Cpx  Multiplication=Matrix(K*u)
  Integrator4 : Integrator  InitialCondition=Y20
  Integrator5 : Integrator  InitialCondition=X20
  Pitch : ToWorkspace  VariableName=Theta2  SampleTime=-1
  PitchRate : ToWorkspace  VariableName=ThetaDot2  SampleTime=-1
  PositionX : ToWorkspace  VariableName=x2  SampleTime=-1
  PositionY : ToWorkspace  VariableName=y2  SampleTime=-1
  Roll : ToWorkspace  VariableName=Psi2  SampleTime=-1
  RollRate : ToWorkspace  VariableName=PsiDot2  SampleTime=-1
  To Workspace1 : ToWorkspace  VariableName=RollReference2  SampleTime=-1
  To Workspace5 : ToWorkspace  VariableName=PitchReference2  SampleTime=-1
  VelocityX : ToWorkspace  VariableName=vx2  SampleTime=-1
  VelocityY : ToWorkspace  VariableName=vy2  SampleTime=-1
  Vx : Outport
  x : Outport  Port=2
  Vy : Outport  Port=3
  y : Outport  Port=4
  wires:
  Demux/1 -> PositionY/1
  Demux1/2 -> VelocityX/1
  Demux1/4 -> RollRate/1
  Demux1/3 -> Roll/1
  Gain4/1 -> Vx/1
  "InputForceY* "/1 -> Gain/1, To Workspace5/1
  Gain/1 -> Add/1
  Demux/4 -> PitchRate/1
  Demux/3 -> Pitch/1
  Add/1 -> Integrator4/1
  Demux1/1 -> PositionX/1
  Gain1/1 -> Vy/1
  InputForceX*/1 -> Gain3/1, To Workspace1/1
  Gain7/1 -> x/1
  Integrator4/1 -> Gain6/1, Gain2/1, Demux/1, Gain1/1
  Demux/2 -> VelocityY/1
  Gain6/1 -> y/1
  Gain3/1 -> Add1/1
  Add1/1 -> Integrator5/1
  Gain2/1 -> Add/2
  Integrator5/1 -> Gain4/1, Gain5/1, Gain7/1, Demux1/1
  Gain5/1 -> Add1/2

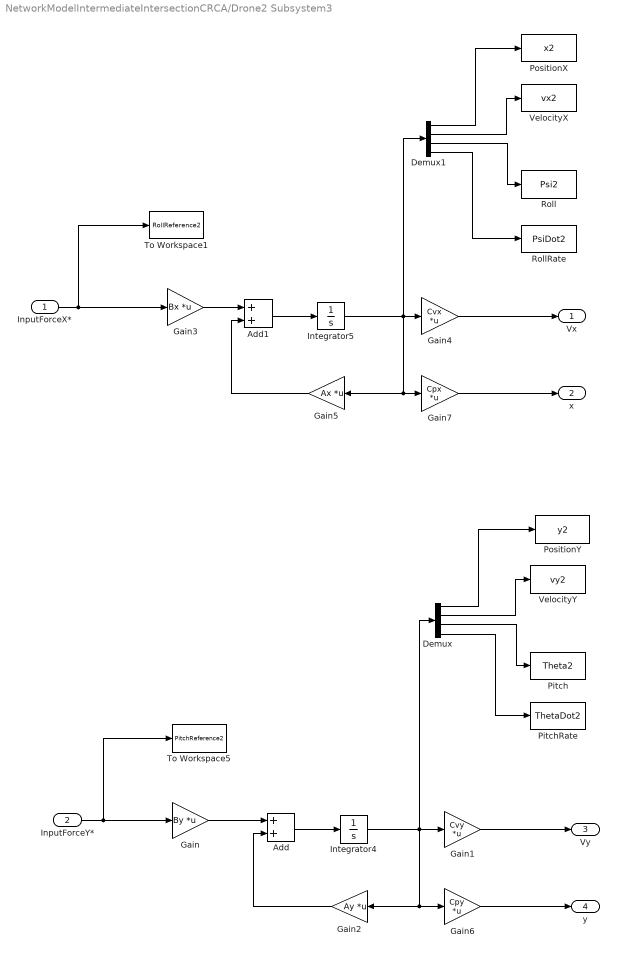
== system NetworkModelIntermediateIntersectionCRCA/Drone2 Subsystem3 ==
  InputForceX* : Inport
  "InputForceY* " : Inport  Port=2
  Add : Sum
  Add1 : Sum
  Demux : Demux
  Demux1 : Demux
  Gain : Gain  Gain=By  Multiplication=Matrix(K*u)
  Gain1 : Gain  Gain=Cvy  Multiplication=Matrix(K*u)
  Gain2 : Gain  Gain=Ay  Multiplication=Matrix(K*u)
  Gain3 : Gain  Gain=Bx  Multiplication=Matrix(K*u)
  Gain4 : Gain  Gain=Cvx  Multiplication=Matrix(K*u)
  Gain5 : Gain  Gain=Ax  Multiplication=Matrix(K*u)
  Gain6 : Gain  Gain=Cpy  Multiplication=Matrix(K*u)
  Gain7 : Gain  Gain=Cpx  Multiplication=Matrix(K*u)
  Integrator4 : Integrator  InitialCondition=Y70
  Integrator5 : Integrator  InitialCondition=X70
  Pitch : ToWorkspace  VariableName=Theta2  SampleTime=-1
  PitchRate : ToWorkspace  VariableName=ThetaDot2  SampleTime=-1
  PositionX : ToWorkspace  VariableName=x2  SampleTime=-1
  PositionY : ToWorkspace  VariableName=y2  SampleTime=-1
  Roll : ToWorkspace  VariableName=Psi2  SampleTime=-1
  RollRate : ToWorkspace  VariableName=PsiDot2  SampleTime=-1
  To Workspace1 : ToWorkspace  VariableName=RollReference2  SampleTime=-1
  To Workspace5 : ToWorkspace  VariableName=PitchReference2  SampleTime=-1
  VelocityX : ToWorkspace  VariableName=vx2  SampleTime=-1
  VelocityY : ToWorkspace  VariableName=vy2  SampleTime=-1
  Vx : Outport
  x : Outport  Port=2
  Vy : Outport  Port=3
  y : Outport  Port=4
  wires:
  Demux/1 -> PositionY/1
  Demux1/2 -> VelocityX/1
  Demux1/4 -> RollRate/1
  Demux1/3 -> Roll/1
  Gain4/1 -> Vx/1
  "InputForceY* "/1 -> Gain/1, To Workspace5/1
  Gain/1 -> Add/1
  Demux/4 -> PitchRate/1
  Demux/3 -> Pitch/1
  Add/1 -> Integrator4/1
  Demux1/1 -> PositionX/1
  Gain1/1 -> Vy/1
  InputForceX*/1 -> Gain3/1, To Workspace1/1
  Gain7/1 -> x/1
  Integrator4/1 -> Gain6/1, Gain2/1, Demux/1, Gain1/1
  Demux/2 -> VelocityY/1
  Gain6/1 -> y/1
  Gain3/1 -> Add1/1
  Add1/1 -> Integrator5/1
  Gain2/1 -> Add/2
  Integrator5/1 -> Gain4/1, Gain5/1, Gain7/1, Demux1/1
  Gain5/1 -> Add1/2

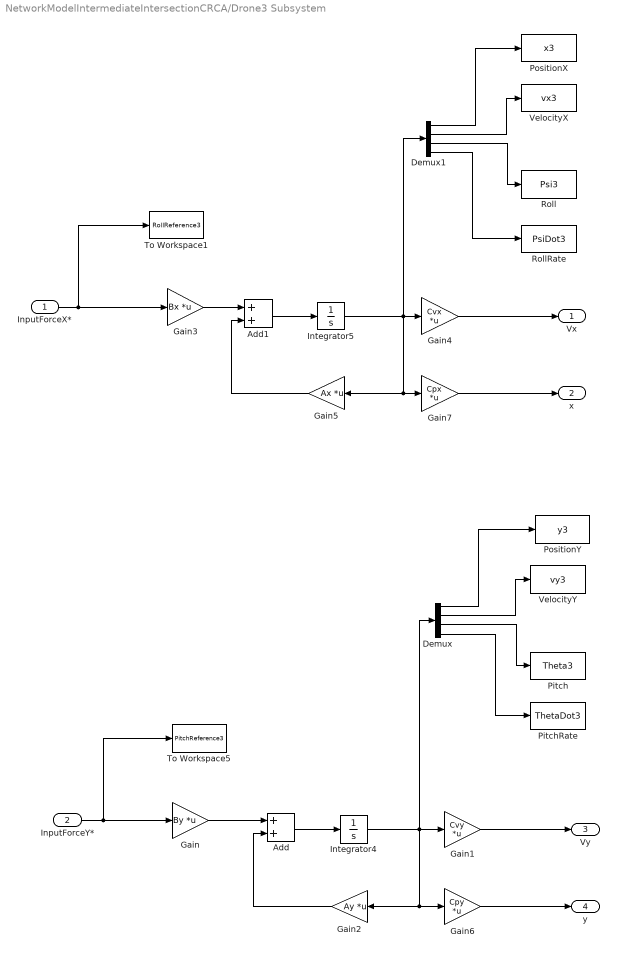
== system NetworkModelIntermediateIntersectionCRCA/Drone3 Subsystem ==
  InputForceX* : Inport
  "InputForceY* " : Inport  Port=2
  Add : Sum
  Add1 : Sum
  Demux : Demux
  Demux1 : Demux
  Gain : Gain  Gain=By  Multiplication=Matrix(K*u)
  Gain1 : Gain  Gain=Cvy  Multiplication=Matrix(K*u)
  Gain2 : Gain  Gain=Ay  Multiplication=Matrix(K*u)
  Gain3 : Gain  Gain=Bx  Multiplication=Matrix(K*u)
  Gain4 : Gain  Gain=Cvx  Multiplication=Matrix(K*u)
  Gain5 : Gain  Gain=Ax  Multiplication=Matrix(K*u)
  Gain6 : Gain  Gain=Cpy  Multiplication=Matrix(K*u)
  Gain7 : Gain  Gain=Cpx  Multiplication=Matrix(K*u)
  Integrator4 : Integrator  InitialCondition=Y30
  Integrator5 : Integrator  InitialCondition=X30
  Pitch : ToWorkspace  VariableName=Theta3  SampleTime=-1
  PitchRate : ToWorkspace  VariableName=ThetaDot3  SampleTime=-1
  PositionX : ToWorkspace  VariableName=x3  SampleTime=-1
  PositionY : ToWorkspace  VariableName=y3  SampleTime=-1
  Roll : ToWorkspace  VariableName=Psi3  SampleTime=-1
  RollRate : ToWorkspace  VariableName=PsiDot3  SampleTime=-1
  To Workspace1 : ToWorkspace  VariableName=RollReference3  SampleTime=-1
  To Workspace5 : ToWorkspace  VariableName=PitchReference3  SampleTime=-1
  VelocityX : ToWorkspace  VariableName=vx3  SampleTime=-1
  VelocityY : ToWorkspace  VariableName=vy3  SampleTime=-1
  Vx : Outport
  x : Outport  Port=2
  Vy : Outport  Port=3
  y : Outport  Port=4
  wires:
  Gain4/1 -> Vx/1
  Demux/2 -> VelocityY/1
  Demux/4 -> PitchRate/1
  Gain3/1 -> Add1/1
  InputForceX*/1 -> Gain3/1, To Workspace1/1
  Gain2/1 -> Add/2
  Demux1/3 -> Roll/1
  Gain7/1 -> x/1
  Add1/1 -> Integrator5/1
  Demux/3 -> Pitch/1
  Gain5/1 -> Add1/2
  Gain6/1 -> y/1
  Integrator5/1 -> Gain4/1, Gain5/1, Gain7/1, Demux1/1
  Gain/1 -> Add/1
  Demux/1 -> PositionY/1
  Add/1 -> Integrator4/1
  Demux1/4 -> RollRate/1
  "InputForceY* "/1 -> Gain/1, To Workspace5/1
  Integrator4/1 -> Gain6/1, Gain2/1, Demux/1, Gain1/1
  Demux1/1 -> PositionX/1
  Demux1/2 -> VelocityX/1
  Gain1/1 -> Vy/1

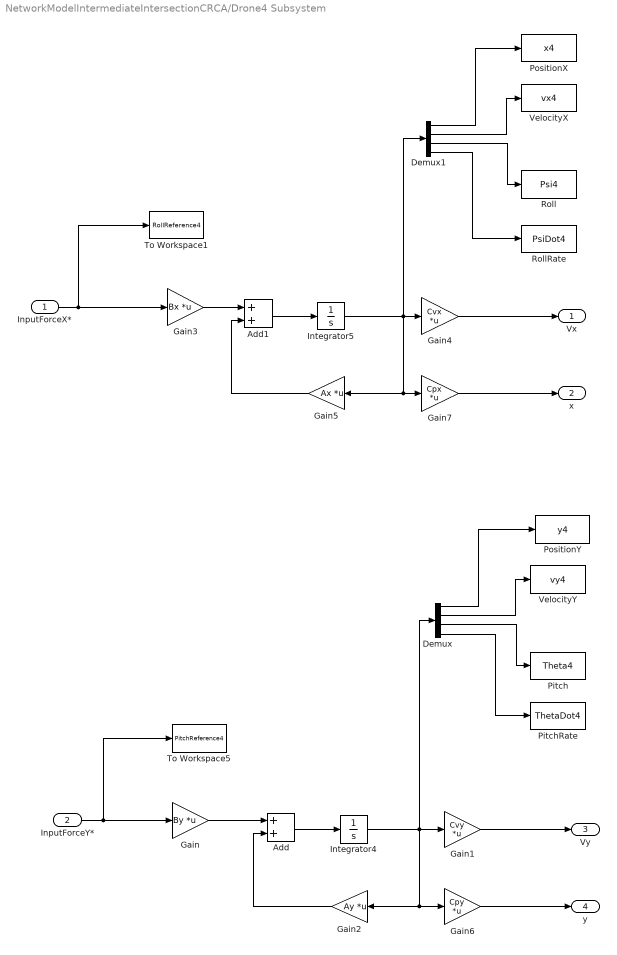
== system NetworkModelIntermediateIntersectionCRCA/Drone4 Subsystem ==
  InputForceX* : Inport
  "InputForceY* " : Inport  Port=2
  Add : Sum
  Add1 : Sum
  Demux : Demux
  Demux1 : Demux
  Gain : Gain  Gain=By  Multiplication=Matrix(K*u)
  Gain1 : Gain  Gain=Cvy  Multiplication=Matrix(K*u)
  Gain2 : Gain  Gain=Ay  Multiplication=Matrix(K*u)
  Gain3 : Gain  Gain=Bx  Multiplication=Matrix(K*u)
  Gain4 : Gain  Gain=Cvx  Multiplication=Matrix(K*u)
  Gain5 : Gain  Gain=Ax  Multiplication=Matrix(K*u)
  Gain6 : Gain  Gain=Cpy  Multiplication=Matrix(K*u)
  Gain7 : Gain  Gain=Cpx  Multiplication=Matrix(K*u)
  Integrator4 : Integrator  InitialCondition=Y40
  Integrator5 : Integrator  InitialCondition=X40
  Pitch : ToWorkspace  VariableName=Theta4  SampleTime=-1
  PitchRate : ToWorkspace  VariableName=ThetaDot4  SampleTime=-1
  PositionX : ToWorkspace  VariableName=x4  SampleTime=-1
  PositionY : ToWorkspace  VariableName=y4  SampleTime=-1
  Roll : ToWorkspace  VariableName=Psi4  SampleTime=-1
  RollRate : ToWorkspace  VariableName=PsiDot4  SampleTime=-1
  To Workspace1 : ToWorkspace  VariableName=RollReference4  SampleTime=-1
  To Workspace5 : ToWorkspace  VariableName=PitchReference4  SampleTime=-1
  VelocityX : ToWorkspace  VariableName=vx4  SampleTime=-1
  VelocityY : ToWorkspace  VariableName=vy4  SampleTime=-1
  Vx : Outport
  x : Outport  Port=2
  Vy : Outport  Port=3
  y : Outport  Port=4
  wires:
  Gain4/1 -> Vx/1
  Demux/2 -> VelocityY/1
  Demux/4 -> PitchRate/1
  Gain3/1 -> Add1/1
  InputForceX*/1 -> Gain3/1, To Workspace1/1
  Gain2/1 -> Add/2
  Demux1/3 -> Roll/1
  Gain7/1 -> x/1
  Add1/1 -> Integrator5/1
  Demux/3 -> Pitch/1
  Gain5/1 -> Add1/2
  Gain6/1 -> y/1
  Integrator5/1 -> Gain4/1, Gain5/1, Gain7/1, Demux1/1
  Gain/1 -> Add/1
  Demux/1 -> PositionY/1
  Add/1 -> Integrator4/1
  Demux1/4 -> RollRate/1
  "InputForceY* "/1 -> Gain/1, To Workspace5/1
  Integrator4/1 -> Gain6/1, Gain2/1, Demux/1, Gain1/1
  Demux1/1 -> PositionX/1
  Demux1/2 -> VelocityX/1
  Gain1/1 -> Vy/1

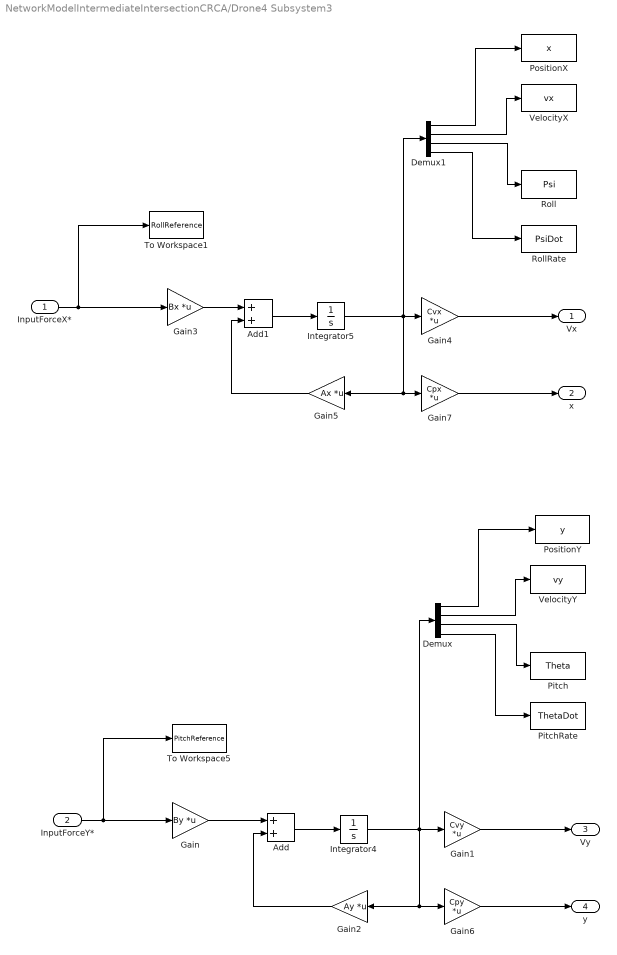
== system NetworkModelIntermediateIntersectionCRCA/Drone4 Subsystem3 ==
  InputForceX* : Inport
  "InputForceY* " : Inport  Port=2
  Add : Sum
  Add1 : Sum
  Demux : Demux
  Demux1 : Demux
  Gain : Gain  Gain=By  Multiplication=Matrix(K*u)
  Gain1 : Gain  Gain=Cvy  Multiplication=Matrix(K*u)
  Gain2 : Gain  Gain=Ay  Multiplication=Matrix(K*u)
  Gain3 : Gain  Gain=Bx  Multiplication=Matrix(K*u)
  Gain4 : Gain  Gain=Cvx  Multiplication=Matrix(K*u)
  Gain5 : Gain  Gain=Ax  Multiplication=Matrix(K*u)
  Gain6 : Gain  Gain=Cpy  Multiplication=Matrix(K*u)
  Gain7 : Gain  Gain=Cpx  Multiplication=Matrix(K*u)
  Integrator4 : Integrator  InitialCondition=Y80
  Integrator5 : Integrator  InitialCondition=X80
  Pitch : ToWorkspace  VariableName=Theta  SampleTime=-1
  PitchRate : ToWorkspace  VariableName=ThetaDot  SampleTime=-1
  PositionX : ToWorkspace  VariableName=x  SampleTime=-1
  PositionY : ToWorkspace  VariableName=y  SampleTime=-1
  Roll : ToWorkspace  VariableName=Psi  SampleTime=-1
  RollRate : ToWorkspace  VariableName=PsiDot  SampleTime=-1
  To Workspace1 : ToWorkspace  VariableName=RollReference  SampleTime=-1
  To Workspace5 : ToWorkspace  VariableName=PitchReference  SampleTime=-1
  VelocityX : ToWorkspace  VariableName=vx  SampleTime=-1
  VelocityY : ToWorkspace  VariableName=vy  SampleTime=-1
  Vx : Outport
  x : Outport  Port=2
  Vy : Outport  Port=3
  y : Outport  Port=4
  wires:
  Gain4/1 -> Vx/1
  Demux/2 -> VelocityY/1
  Demux/4 -> PitchRate/1
  Gain3/1 -> Add1/1
  InputForceX*/1 -> Gain3/1, To Workspace1/1
  Gain2/1 -> Add/2
  Demux1/3 -> Roll/1
  Gain7/1 -> x/1
  Add1/1 -> Integrator5/1
  Demux/3 -> Pitch/1
  Gain5/1 -> Add1/2
  Gain6/1 -> y/1
  Integrator5/1 -> Gain4/1, Gain5/1, Gain7/1, Demux1/1
  Gain/1 -> Add/1
  Demux/1 -> PositionY/1
  Add/1 -> Integrator4/1
  Demux1/4 -> RollRate/1
  "InputForceY* "/1 -> Gain/1, To Workspace5/1
  Integrator4/1 -> Gain6/1, Gain2/1, Demux/1, Gain1/1
  Demux1/1 -> PositionX/1
  Demux1/2 -> VelocityX/1
  Gain1/1 -> Vy/1

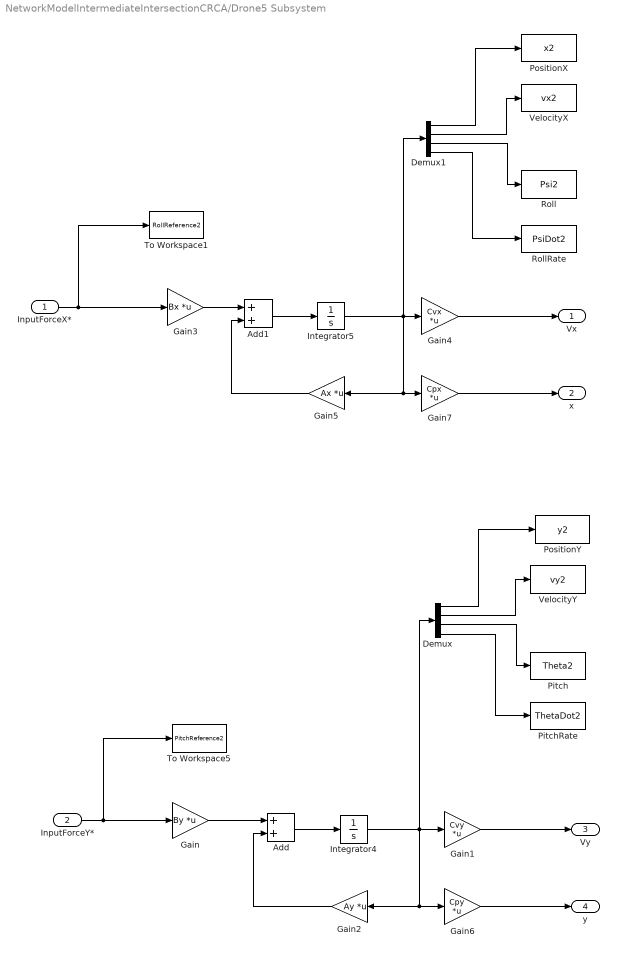
== system NetworkModelIntermediateIntersectionCRCA/Drone5 Subsystem ==
  InputForceX* : Inport
  "InputForceY* " : Inport  Port=2
  Add : Sum
  Add1 : Sum
  Demux : Demux
  Demux1 : Demux
  Gain : Gain  Gain=By  Multiplication=Matrix(K*u)
  Gain1 : Gain  Gain=Cvy  Multiplication=Matrix(K*u)
  Gain2 : Gain  Gain=Ay  Multiplication=Matrix(K*u)
  Gain3 : Gain  Gain=Bx  Multiplication=Matrix(K*u)
  Gain4 : Gain  Gain=Cvx  Multiplication=Matrix(K*u)
  Gain5 : Gain  Gain=Ax  Multiplication=Matrix(K*u)
  Gain6 : Gain  Gain=Cpy  Multiplication=Matrix(K*u)
  Gain7 : Gain  Gain=Cpx  Multiplication=Matrix(K*u)
  Integrator4 : Integrator  InitialCondition=Y50
  Integrator5 : Integrator  InitialCondition=X50
  Pitch : ToWorkspace  VariableName=Theta2  SampleTime=-1
  PitchRate : ToWorkspace  VariableName=ThetaDot2  SampleTime=-1
  PositionX : ToWorkspace  VariableName=x2  SampleTime=-1
  PositionY : ToWorkspace  VariableName=y2  SampleTime=-1
  Roll : ToWorkspace  VariableName=Psi2  SampleTime=-1
  RollRate : ToWorkspace  VariableName=PsiDot2  SampleTime=-1
  To Workspace1 : ToWorkspace  VariableName=RollReference2  SampleTime=-1
  To Workspace5 : ToWorkspace  VariableName=PitchReference2  SampleTime=-1
  VelocityX : ToWorkspace  VariableName=vx2  SampleTime=-1
  VelocityY : ToWorkspace  VariableName=vy2  SampleTime=-1
  Vx : Outport
  x : Outport  Port=2
  Vy : Outport  Port=3
  y : Outport  Port=4
  wires:
  Demux/1 -> PositionY/1
  Demux1/2 -> VelocityX/1
  Demux1/4 -> RollRate/1
  Demux1/3 -> Roll/1
  Gain4/1 -> Vx/1
  "InputForceY* "/1 -> Gain/1, To Workspace5/1
  Gain/1 -> Add/1
  Demux/4 -> PitchRate/1
  Demux/3 -> Pitch/1
  Add/1 -> Integrator4/1
  Demux1/1 -> PositionX/1
  Gain1/1 -> Vy/1
  InputForceX*/1 -> Gain3/1, To Workspace1/1
  Gain7/1 -> x/1
  Integrator4/1 -> Gain6/1, Gain2/1, Demux/1, Gain1/1
  Demux/2 -> VelocityY/1
  Gain6/1 -> y/1
  Gain3/1 -> Add1/1
  Add1/1 -> Integrator5/1
  Gain2/1 -> Add/2
  Integrator5/1 -> Gain4/1, Gain5/1, Gain7/1, Demux1/1
  Gain5/1 -> Add1/2

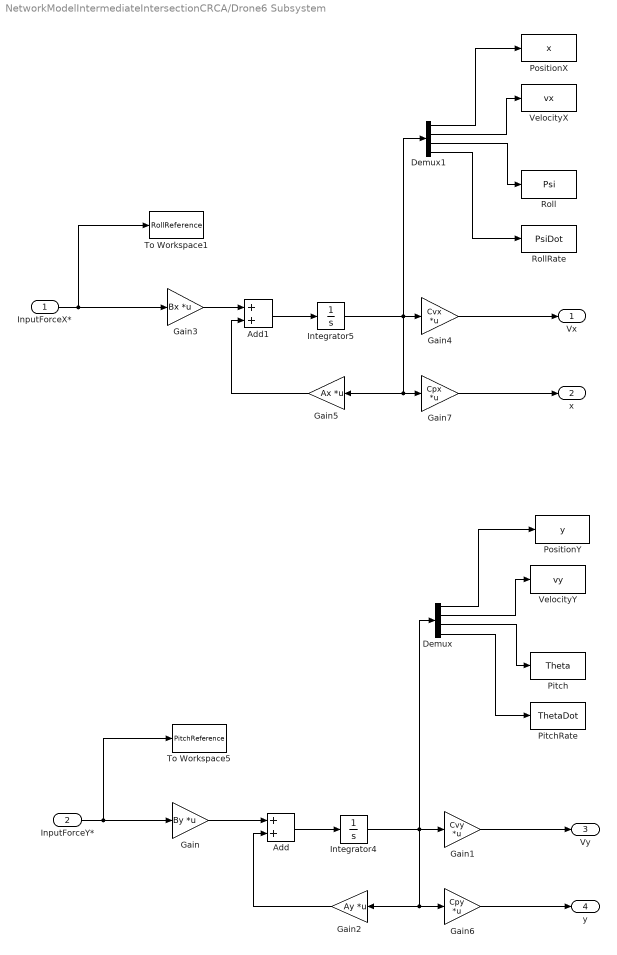
== system NetworkModelIntermediateIntersectionCRCA/Drone6 Subsystem ==
  InputForceX* : Inport
  "InputForceY* " : Inport  Port=2
  Add : Sum
  Add1 : Sum
  Demux : Demux
  Demux1 : Demux
  Gain : Gain  Gain=By  Multiplication=Matrix(K*u)
  Gain1 : Gain  Gain=Cvy  Multiplication=Matrix(K*u)
  Gain2 : Gain  Gain=Ay  Multiplication=Matrix(K*u)
  Gain3 : Gain  Gain=Bx  Multiplication=Matrix(K*u)
  Gain4 : Gain  Gain=Cvx  Multiplication=Matrix(K*u)
  Gain5 : Gain  Gain=Ax  Multiplication=Matrix(K*u)
  Gain6 : Gain  Gain=Cpy  Multiplication=Matrix(K*u)
  Gain7 : Gain  Gain=Cpx  Multiplication=Matrix(K*u)
  Integrator4 : Integrator  InitialCondition=Y60
  Integrator5 : Integrator  InitialCondition=X60
  Pitch : ToWorkspace  VariableName=Theta  SampleTime=-1
  PitchRate : ToWorkspace  VariableName=ThetaDot  SampleTime=-1
  PositionX : ToWorkspace  VariableName=x  SampleTime=-1
  PositionY : ToWorkspace  VariableName=y  SampleTime=-1
  Roll : ToWorkspace  VariableName=Psi  SampleTime=-1
  RollRate : ToWorkspace  VariableName=PsiDot  SampleTime=-1
  To Workspace1 : ToWorkspace  VariableName=RollReference  SampleTime=-1
  To Workspace5 : ToWorkspace  VariableName=PitchReference  SampleTime=-1
  VelocityX : ToWorkspace  VariableName=vx  SampleTime=-1
  VelocityY : ToWorkspace  VariableName=vy  SampleTime=-1
  Vx : Outport
  x : Outport  Port=2
  Vy : Outport  Port=3
  y : Outport  Port=4
  wires:
  Gain4/1 -> Vx/1
  Demux/2 -> VelocityY/1
  Demux/4 -> PitchRate/1
  Gain3/1 -> Add1/1
  InputForceX*/1 -> Gain3/1, To Workspace1/1
  Gain2/1 -> Add/2
  Demux1/3 -> Roll/1
  Gain7/1 -> x/1
  Add1/1 -> Integrator5/1
  Demux/3 -> Pitch/1
  Gain5/1 -> Add1/2
  Gain6/1 -> y/1
  Integrator5/1 -> Gain4/1, Gain5/1, Gain7/1, Demux1/1
  Gain/1 -> Add/1
  Demux/1 -> PositionY/1
  Add/1 -> Integrator4/1
  Demux1/4 -> RollRate/1
  "InputForceY* "/1 -> Gain/1, To Workspace5/1
  Integrator4/1 -> Gain6/1, Gain2/1, Demux/1, Gain1/1
  Demux1/1 -> PositionX/1
  Demux1/2 -> VelocityX/1
  Gain1/1 -> Vy/1

== system NetworkModelIntermediateIntersectionCRCA/If Action Subsystem1 ==
  deltaVx5 : Inport
  deltaVy5 : Inport  Port=2
  Action Port : ActionPort  ActionType=then
  dVx5 : Outport
  dVy5 : Outport  Port=2
  wires:
  deltaVx5/1 -> dVx5/1
  deltaVy5/1 -> dVy5/1

== system NetworkModelIntermediateIntersectionCRCA/If Action Subsystem2 ==
  deltaVx2 : Inport
  deltaVy2 : Inport  Port=2
  Action Port : ActionPort  ActionType=then
  dVx2 : Outport
  dVy2 : Outport  Port=2
  wires:
  deltaVx2/1 -> dVx2/1
  deltaVy2/1 -> dVy2/1

== system NetworkModelIntermediateIntersectionCRCA/If Action Subsystem3 ==
  deltaVx4 : Inport
  deltaVy4 : Inport  Port=2
  Action Port : ActionPort  ActionType=then
  dVx4 : Outport
  dVy4 : Outport  Port=2
  wires:
  deltaVx4/1 -> dVx4/1
  deltaVy4/1 -> dVy4/1

== system NetworkModelIntermediateIntersectionCRCA/If Action Subsystem4 ==
  deltaVx6 : Inport
  deltaVy6 : Inport  Port=2
  Action Port : ActionPort  ActionType=then
  dVx6 : Outport
  dVy6 : Outport  Port=2
  wires:
  deltaVx6/1 -> dVx6/1
  deltaVy6/1 -> dVy6/1

== system NetworkModelIntermediateIntersectionCRCA/If Action Subsystem5 ==
  deltaVx1 : Inport
  deltaVy1 : Inport  Port=2
  Action Port : ActionPort  ActionType=then
  dVx1 : Outport
  dVy1 : Outport  Port=2
  wires:
  deltaVx1/1 -> dVx1/1
  deltaVy1/1 -> dVy1/1

== system NetworkModelIntermediateIntersectionCRCA/If Action Subsystem6 ==
  deltaVx3 : Inport
  deltaVy3 : Inport  Port=2
  Action Port : ActionPort  ActionType=then
  dVx3 : Outport
  dVy3 : Outport  Port=2
  wires:
  deltaVx3/1 -> dVx3/1
  deltaVy3/1 -> dVy3/1

== system NetworkModelIntermediateIntersectionCRCA/If Action Subsystem7 ==
  deltaVx7 : Inport
  deltaVy7 : Inport  Port=2
  Action Port : ActionPort  ActionType=then
  dVx7 : Outport
  dVy7 : Outport  Port=2
  wires:
  deltaVx7/1 -> dVx7/1
  deltaVy7/1 -> dVy7/1

== system NetworkModelIntermediateIntersectionCRCA/If Action Subsystem8 ==
  deltaVx8 : Inport
  deltaVy8 : Inport  Port=2
  Action Port : ActionPort  ActionType=then
  dVx8 : Outport
  dVy8 : Outport  Port=2
  wires:
  deltaVx8/1 -> dVx8/1
  deltaVy8/1 -> dVy8/1

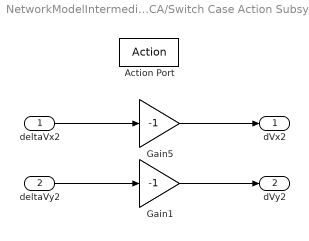
== system NetworkModelIntermediateIntersectionCRCA/Switch Case Action Subsystem ==
  deltaVx2 : Inport
  deltaVy2 : Inport  Port=2
  Action Port : ActionPort  ActionType=elseif
  Gain1 : Gain  Gain=-1
  Gain5 : Gain  Gain=-1
  dVx2 : Outport
  dVy2 : Outport  Port=2
  wires:
  deltaVy2/1 -> Gain1/1
  deltaVx2/1 -> Gain5/1
  Gain5/1 -> dVx2/1
  Gain1/1 -> dVy2/1

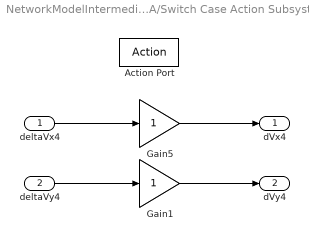
== system NetworkModelIntermediateIntersectionCRCA/Switch Case Action Subsystem1 ==
  deltaVx4 : Inport
  deltaVy4 : Inport  Port=2
  Action Port : ActionPort  ActionType=elseif
  Gain1 : Gain
  Gain5 : Gain
  dVx4 : Outport
  dVy4 : Outport  Port=2
  wires:
  deltaVy4/1 -> Gain1/1
  deltaVx4/1 -> Gain5/1
  Gain5/1 -> dVx4/1
  Gain1/1 -> dVy4/1

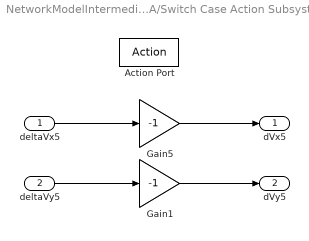
== system NetworkModelIntermediateIntersectionCRCA/Switch Case Action Subsystem2 ==
  deltaVx5 : Inport
  deltaVy5 : Inport  Port=2
  Action Port : ActionPort  ActionType=elseif
  Gain1 : Gain  Gain=-1
  Gain5 : Gain  Gain=-1
  dVx5 : Outport
  dVy5 : Outport  Port=2
  wires:
  deltaVy5/1 -> Gain1/1
  deltaVx5/1 -> Gain5/1
  Gain5/1 -> dVx5/1
  Gain1/1 -> dVy5/1

== system NetworkModelIntermediateIntersectionCRCA/Switch Case Action Subsystem3 ==
  deltaVx6 : Inport
  deltaVy6 : Inport  Port=2
  Action Port : ActionPort  ActionType=elseif
  Gain1 : Gain
  Gain5 : Gain
  dVx6 : Outport
  dVy6 : Outport  Port=2
  wires:
  deltaVy6/1 -> Gain1/1
  deltaVx6/1 -> Gain5/1
  Gain5/1 -> dVx6/1
  Gain1/1 -> dVy6/1

== system NetworkModelIntermediateIntersectionCRCA/Switch Case Action Subsystem4 ==
  deltaVx1 : Inport
  deltaVy1 : Inport  Port=2
  Action Port : ActionPort  ActionType=elseif
  Gain1 : Gain  Gain=-1
  Gain5 : Gain  Gain=-1
  dVx1 : Outport
  dVy1 : Outport  Port=2
  wires:
  deltaVy1/1 -> Gain1/1
  deltaVx1/1 -> Gain5/1
  Gain5/1 -> dVx1/1
  Gain1/1 -> dVy1/1

== system NetworkModelIntermediateIntersectionCRCA/Switch Case Action Subsystem5 ==
  deltaVx3 : Inport
  deltaVy3 : Inport  Port=2
  Action Port : ActionPort  ActionType=elseif
  Gain1 : Gain
  Gain5 : Gain
  dVx3 : Outport
  dVy3 : Outport  Port=2
  wires:
  deltaVy3/1 -> Gain1/1
  deltaVx3/1 -> Gain5/1
  Gain5/1 -> dVx3/1
  Gain1/1 -> dVy3/1

== system NetworkModelIntermediateIntersectionCRCA/Switch Case Action Subsystem6 ==
  deltaVx7 : Inport
  deltaVy7 : Inport  Port=2
  Action Port : ActionPort  ActionType=elseif
  Gain1 : Gain  Gain=-1
  Gain5 : Gain  Gain=-1
  dVx7 : Outport
  dVy7 : Outport  Port=2
  wires:
  deltaVy7/1 -> Gain1/1
  deltaVx7/1 -> Gain5/1
  Gain5/1 -> dVx7/1
  Gain1/1 -> dVy7/1

== system NetworkModelIntermediateIntersectionCRCA/Switch Case Action Subsystem7 ==
  deltaVx4 : Inport
  deltaVy4 : Inport  Port=2
  Action Port : ActionPort  ActionType=elseif
  Gain1 : Gain
  Gain5 : Gain
  dVx4 : Outport
  dVy4 : Outport  Port=2
  wires:
  deltaVy4/1 -> Gain1/1
  deltaVx4/1 -> Gain5/1
  Gain5/1 -> dVx4/1
  Gain1/1 -> dVy4/1

== matlab function NetworkModelIntermediateIntersectionCRCA/MATLAB Function1 ==
  data: qDotxi input; y output; qDotxj input; qDotyi input; qDotyj input
function y = ClosureRate(qDotxi, qDotxj, qDotyi, qDotyj)

Vmax = 0.2;
K = 1;
Vdiff = K*sqrt((qDotxi - qDotxj)^2 + (qDotyi - qDotyj)^2); 

if abs(Vdiff)>=Vmax/2
    Vdiff = Vmax/2;
end 

y = Vdiff;
